simulink model "Hermes"  (R2022a)
settings: Solver=FixedStepAuto  StartTime=0.0  StopTime=10.0  FixedStep=0.005  RelTol=1e-3
values from neighbouring files (symbols this model uses):
  Car_mass = Car_Mass_lb * 0.45359    (= 272.154)    [hermes_physical_parameters.m]    (also in hermes_physical_parameters.mat; input_signals.mat)
  Car_moment_of_inertia = 4 * (0.06631756 + 0.06646249)    (= 0.5311202)    [hermes_physical_parameters.m]    (also in hermes_physical_parameters.mat; input_signals.mat)
  Cross_sectional_area = 0.78    [hermes_physical_parameters.m]    (also in hermes_physical_parameters.mat; input_signals.mat)
  DIFF_ratio = 9    [datasheet.mat]    (also in hermes_system_parameters.m = 8.38; hermes_system_parameters.mat = 8.38; input_signals.mat = 8.38)
  Drag_coeff = 0.5    [datasheet.mat]    (also in hermes_physical_parameters.m = 0.906; hermes_physical_parameters.mat = 0.906; input_signals.mat = 0.906)
  ECVT_angle = 13    [hermes_system_parameters.m]    (also in hermes_system_parameters.mat; input_signals.mat)
  ECVT_clamp_gain = 0.0001    [datasheet.mat]    (also in hermes_system_parameters.m = 0.001; hermes_system_parameters.mat = 0.001; input_signals.mat = 0.0006)
  ECVT_efficiency = 0.8    [datasheet.mat]    (also in hermes_physical_parameters.m = 0.88; hermes_physical_parameters.mat = 0.88; input_signals.mat = 0.88)
  ECVT_friction_coeff = 0.51    [hermes_physical_parameters.m]    (also in hermes_physical_parameters.mat; input_signals.mat)
  ECVT_max_clamp_force = ECVT_max_clamp_force * 4.4482189    (= 889.64378)    [hermes_system_parameters.m]    (also in hermes_system_parameters.mat; input_signals.mat)
  ECVT_MAX_ratio = 4.24    [datasheet.mat]    (also in hermes_system_parameters.m = 4.31; hermes_system_parameters.mat = 4.31; input_signals.mat = 4.31)
  ECVT_MIN_ratio = 0.81    [datasheet.mat]    (also in hermes_system_parameters.m; hermes_system_parameters.mat; input_signals.mat)
  ECVT_P_gain = 7e-05    [datasheet.mat]    (also in hermes_system_parameters.m; hermes_system_parameters.mat; input_signals.mat)
  ECVT_rate_limit = (ECVT_MAX_ratio - ECVT_MIN_ratio) / ECVT_shift_time    (= 3.5)    [hermes_system_parameters.m]    (also in hermes_system_parameters.mat; input_signals.mat)
  Engine_efficiency = 0.9    [datasheet.mat]    (also in hermes_physical_parameters.m = 1; hermes_physical_parameters.mat = 1; input_signals.mat = 1)
  Engine_moment_of_inertia = 0.00172765 + 0.03589500    (= 0.03762265)    [hermes_physical_parameters.m]    (also in hermes_physical_parameters.mat; input_signals.mat)
  GRAVITY = 9.81    [datasheet.mat]    (also in hermes_physical_parameters.m; hermes_physical_parameters.mat; input_signals.mat)
  launch_control_enabled = 1    [input_signals.mat]
  Locked_regime_rpm = 3200    [hermes_system_parameters.m]    (also in hermes_system_parameters.mat; input_signals.mat = 3100)
  Rolling_coeff = 0.125    [hermes_physical_parameters.m]    (also in hermes_physical_parameters.mat; input_signals.mat)
  RPM_MAX = 3600    [datasheet.mat]    (also in hermes_physical_parameters.m; hermes_physical_parameters.mat; input_signals.mat)
  RPM_STALL = 1800    [datasheet.mat]    (also in hermes_physical_parameters.m = 2200; hermes_physical_parameters.mat = 2200; input_signals.mat = 2200)
  Slip_regime_rpm = 2400    [hermes_system_parameters.m]    (also in hermes_system_parameters.mat; input_signals.mat = 2800)
  Torque_regime_limit = 10176    [datasheet.mat]
  Transmission_efficiency = 0.95 * 0.95 * 0.95 * 0.95    (= 0.81450625)    [hermes_physical_parameters.m]    (also in hermes_physical_parameters.mat; input_signals.mat)
  Wheel_radius = 0.2921    [datasheet.mat]    (also in hermes_physical_parameters.m; hermes_physical_parameters.mat; input_signals.mat)
undefined symbols (not defined in the file or in its folder): Target_Engine_rpm, Wheel_RPM
libraries: simulink_extras x3, simulink x1
settings Model: Creator=garyw  LastModifiedBy=garyw

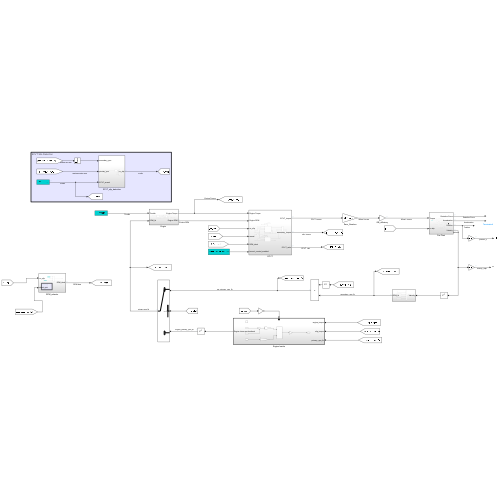
[thumbnail: Simulink's stored preview of the top-level diagram]
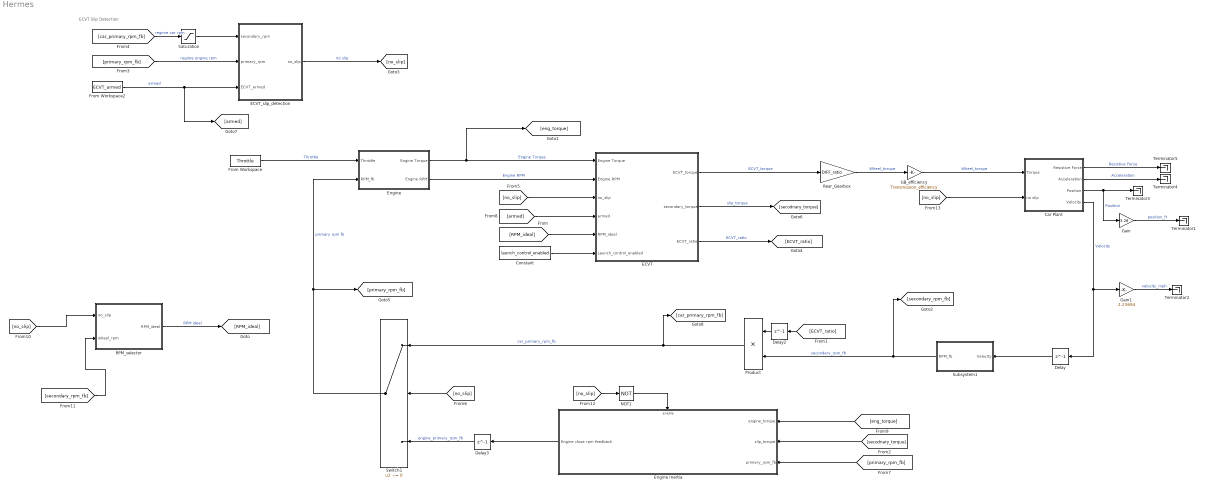
== system Hermes ==
  note: ECVT Slip Detection
  Car Plant : Subsystem
  Constant : Constant  Value=launch_control_enabled
  Delay : Delay  DelayLength=1
  Delay2 : Delay  DelayLength=1  InitialCondition=ECVT_MAX_ratio
  Delay3 : Delay  DelayLength=1  InitialCondition=1800
  ECVT : Subsystem
  ECVT_slip_detection : Subsystem
  Engine : Subsystem
  Engine Inertia : Subsystem
  From Workspace : FromWorkspace  VariableName=Throttle
  From Workspace2 : FromWorkspace  VariableName=ECVT_armed
  GB_efficiency : Gain  Gain=Transmission_efficiency
  Gain : Gain  Gain=3.28
  Gain1 : Gain  Gain=2.23694
  NOT1 : Logic  Operator=NOT  IconShape=distinctive  AllPortsSameDT=off  OutDataTypeStr=boolean
  Product : Product
  RPM_selector : Subsystem
  Rear_Gearbox : Gain  Gain=DIFF_ratio
  Saturation : Saturate  UpperLimit=inf  LowerLimit=0.001
  Subsystem1 : Subsystem
  Switch1 : Switch  Criteria=u2 ~= 0  SaturateOnIntegerOverflow=off  InputSameDT=off
  Terminator{1..5} (5 alike) : Terminator
  wires:
  From Workspace/1 -> Engine/1(Throttle)  "Throttle"
  Engine/1(Engine Torque) -> [eng_torque], ECVT/1(Engine Torque)  "Engine Torque"
  GB_efficiency/1 -> Car Plant/1(Torque)  "Wheel_torque"
  Car Plant/2(Acceleration) -> Terminator4/1  "Acceleration"
  Car Plant/3(Position) -> Terminator3/1, Gain/1  "Position"
  RPM_selector/1(RPM_ideal) -> [RPM_ideal]  "RPM ideal"
  ECVT_slip_detection/1(no_slip) -> [no_slip]  "no slip"
  Subsystem1/1(RPM_fb) -> [secondary_rpm_fb], Product/2  "secondary_rpm_fb"
  Car Plant/4(Velocity) -> Gain1/1, Delay/1  "Velocity"
  [no_slip] -> Switch1/2
  [primary_rpm_fb] -> Engine Inertia/3(primary_rpm_fb)
  [secodnary_torque] -> Engine Inertia/2(slip_torque)
  [eng_torque] -> Engine Inertia/1(engine_torque)
  Switch1/1 -> [primary_rpm_fb], Engine/2(RPM_fb)  "primary rpm fb"
  Product/1 -> [car_primary_rpm_fb], Switch1/1  "car_primary_rpm_fb"
  [ECVT_ratio] -> Delay2/1
  Engine Inertia/1(Engine close rpm feedback) -> Delay3/1
  [no_slip] -> NOT1/1
  NOT1/1 -> Engine Inertia/Enable
  [primary_rpm_fb] -> ECVT_slip_detection/2(primary_rpm)  "regime engine rpm"
  [car_primary_rpm_fb] -> Saturation/1  "regime car rpm"
  Delay/1 -> Subsystem1/1(Velocity)
  Saturation/1 -> ECVT_slip_detection/1(secondary_rpm)
  Delay2/1 -> Product/1
  Delay3/1 -> Switch1/3  "engine_primary_rpm_fb"
  [no_slip] -> Car Plant/2(no slip)
  From Workspace2/1 -> [armed], ECVT_slip_detection/3(ECVT_armed)  "armed"
  Engine/2(Engine RPM) -> ECVT/2(Engine RPM)  "Engine RPM"
  ECVT/1(ECVT_torque) -> Rear_Gearbox/1  "ECVT_torque"
  [RPM_ideal] -> ECVT/5(RPM_ideal)
  ECVT/3(ECVT_ratio) -> [ECVT_ratio]  "ECVT_ratio"
  ECVT/2(secondary_torque) -> [secodnary_torque]  "slip_torque"
  [no_slip] -> ECVT/3(no_slip)
  [armed] -> ECVT/4(armed)
  Rear_Gearbox/1 -> GB_efficiency/1  "Wheel_torque"
  [no_slip] -> RPM_selector/1(no_slip)
  Constant/1 -> ECVT/6(Launch_control_enabled)
  Gain/1 -> Terminator1/1  "position_ft"
  Gain1/1 -> Terminator2/1  "velocity_mph"
  [secondary_rpm_fb] -> RPM_selector/2(wheel_rpm)
  Car Plant/1(Resistive Force) -> Terminator5/1  "Resistive Force"

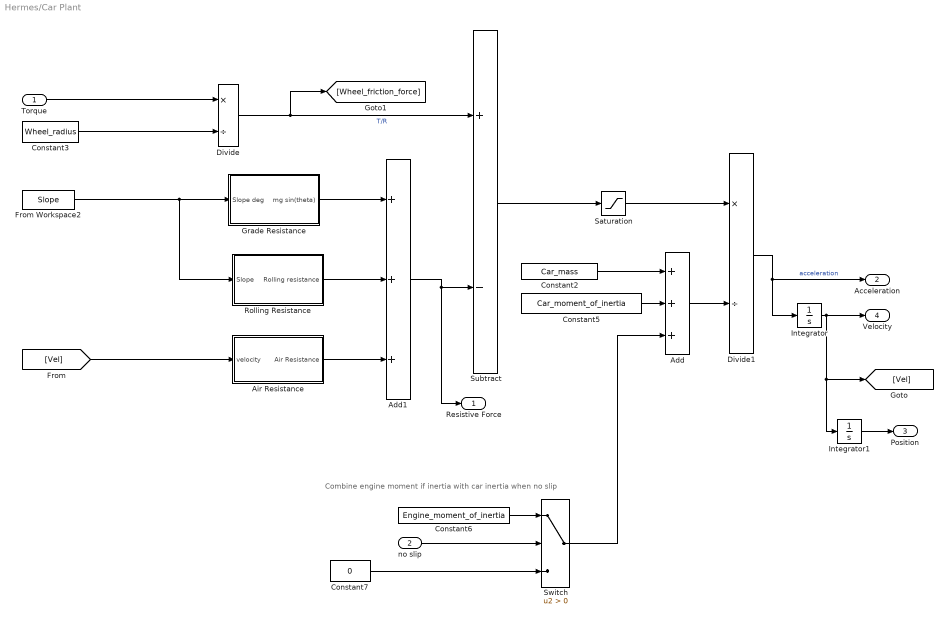
== system Hermes/Car Plant ==
  note: Combine engine moment if inertia with car inertia when no slip
  Torque : Inport
  no slip : Inport  Port=2
  Add : Sum  Inputs=+++
  Add1 : Sum  Inputs=+++
  Air Resistance : Subsystem
  Constant2 : Constant  Value=Car_mass
  Constant3 : Constant  Value=Wheel_radius
  Constant5 : Constant  Value=Car_moment_of_inertia
  Constant6 : Constant  Value=Engine_moment_of_inertia
  Constant7 : Constant  Value=0
  Divide : Product  Inputs=*/
  Divide1 : Product  Inputs=*/
  From Workspace2 : FromWorkspace  VariableName=Slope
  Grade Resistance : Subsystem
  Integrator : Integrator
  Integrator1 : Integrator
  Rolling Resistance : Subsystem
  Saturation : Saturate  UpperLimit=inf  LowerLimit=0
  Subtract : Sum  Inputs=+-
  Switch : Switch  Criteria=u2 > Threshold  SaturateOnIntegerOverflow=off  InputSameDT=off
  Resistive Force : Outport
  Acceleration : Outport  Port=2
  Position : Outport  Port=3
  Velocity : Outport  Port=4
  wires:
  Constant3/1 -> Divide/2
  Divide/1 -> [Wheel_friction_force], Subtract/1  "T/R"
  Subtract/1 -> Saturation/1
  Divide1/1 -> Integrator/1, Acceleration/1  "acceleration"
  Torque/1 -> Divide/1
  Integrator/1 -> [Vel], Integrator1/1, Velocity/1
  Integrator1/1 -> Position/1
  Constant2/1 -> Add/1
  Add/1 -> Divide1/2
  Constant5/1 -> Add/2
  Switch/1 -> Add/3
  Constant6/1 -> Switch/1
  no slip/1 -> Switch/2
  Constant7/1 -> Switch/3
  From Workspace2/1 -> Rolling Resistance/1(Slope), Grade Resistance/1(Slope deg)
  Grade Resistance/1(mg sin(theta)) -> Add1/1
  [Vel] -> Air Resistance/1(velocity)
  Rolling Resistance/1(Rolling resistance) -> Add1/2
  Air Resistance/1(Air Resistance) -> Add1/3
  Saturation/1 -> Divide1/1
  Add1/1 -> Resistive Force/1, Subtract/2

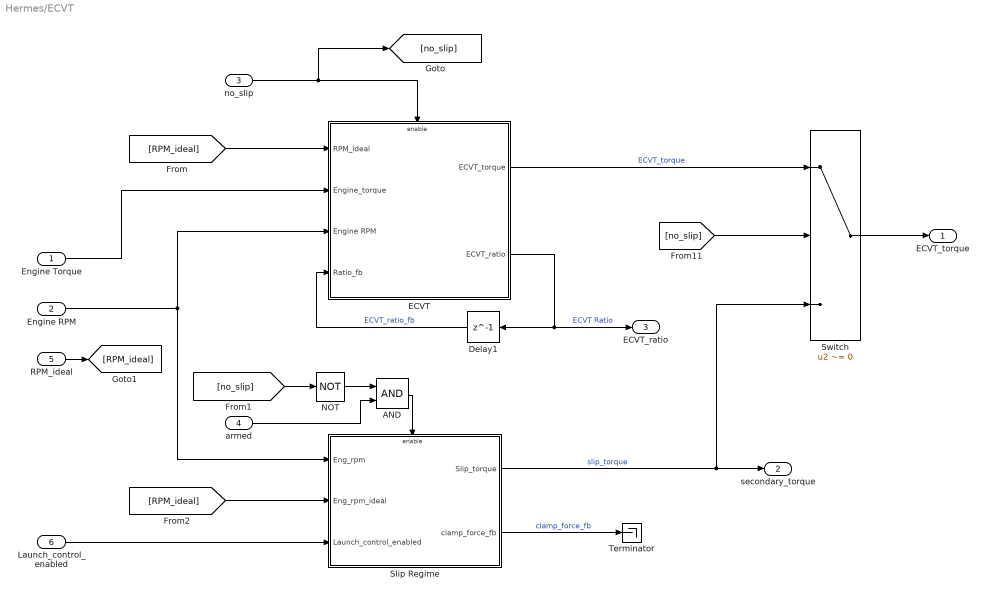
== system Hermes/ECVT ==
  Engine Torque : Inport
  Engine RPM : Inport  Port=2
  no_slip : Inport  Port=3
  armed : Inport  Port=4
  RPM_ideal : Inport  Port=5
  Launch_control_enabled : Inport  Port=6
  AND : Logic  AllPortsSameDT=off  OutDataTypeStr=boolean
  Delay1 : Delay  DelayLength=1  InitialCondition=ECVT_MAX_ratio
  ECVT : Subsystem
  NOT : Logic  Operator=NOT  IconShape=distinctive  AllPortsSameDT=off  OutDataTypeStr=boolean
  Slip Regime : Subsystem
  Switch : Switch  Criteria=u2 ~= 0  SaturateOnIntegerOverflow=off  InputSameDT=off
  Terminator : Terminator
  ECVT_torque : Outport
  secondary_torque : Outport  Port=2
  ECVT_ratio : Outport  Port=3
  wires:
  [RPM_ideal] -> Slip Regime/2(Eng_rpm_ideal)
  ECVT/1(ECVT_torque) -> Switch/1  "ECVT_torque"
  [RPM_ideal] -> ECVT/1(RPM_ideal)
  Slip Regime/1(Slip_torque) -> secondary_torque/1, Switch/3  "slip_torque"
  Delay1/1 -> ECVT/4(Ratio_fb)  "ECVT_ratio_fb"
  Engine RPM/1 -> Slip Regime/1(Eng_rpm), ECVT/3(Engine RPM)
  no_slip/1 -> [no_slip], ECVT/Enable
  [no_slip] -> NOT/1
  ECVT/2(ECVT_ratio) -> ECVT_ratio/1, Delay1/1  "ECVT Ratio"
  NOT/1 -> AND/1
  [no_slip] -> Switch/2
  Slip Regime/2(clamp_force_fb) -> Terminator/1  "clamp_force_fb"
  AND/1 -> Slip Regime/Enable
  armed/1 -> AND/2
  Engine Torque/1 -> ECVT/2(Engine_torque)
  Switch/1 -> ECVT_torque/1
  RPM_ideal/1 -> [RPM_ideal]
  Launch_control_enabled/1 -> Slip Regime/3(Launch_control_enabled)

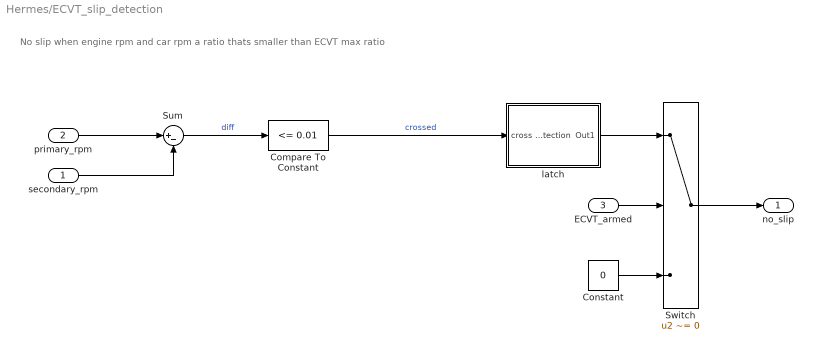
== system Hermes/ECVT_slip_detection ==
  note: No slip when engine rpm and car rpm a ratio thats smaller than ECVT max ratio
  secondary_rpm : Inport
  primary_rpm : Inport  Port=2
  ECVT_armed : Inport  Port=3
  Compare To Constant : simulink/Logic and Bit Operations/Compare To Constant  relop=<=  const=0.01  OutDataTypeStr=boolean
  Constant : Constant  Value=0
  Sum : Sum  Inputs=|+-
  Switch : Switch  Criteria=u2 ~= 0  SaturateOnIntegerOverflow=off  InputSameDT=off
  latch : Subsystem
  no_slip : Outport
  wires:
  secondary_rpm/1 -> Sum/2
  primary_rpm/1 -> Sum/1
  Compare To Constant/1 -> latch/1(cross detection)  "crossed"
  Sum/1 -> Compare To Constant/1  "diff"
  Switch/1 -> no_slip/1
  Constant/1 -> Switch/3
  ECVT_armed/1 -> Switch/2
  latch/1(Out1) -> Switch/1

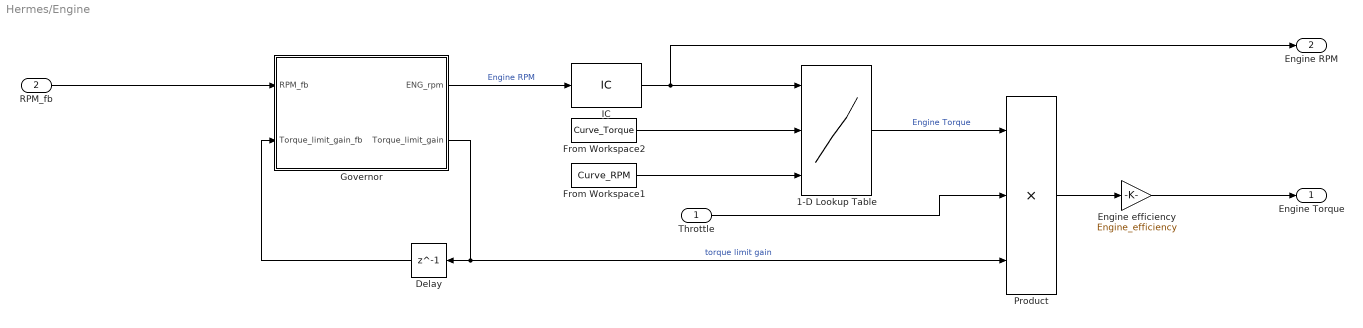
== system Hermes/Engine ==
  Throttle : Inport
  RPM_fb : Inport  Port=2
  1-D Lookup Table : Lookup_n-D  NumberOfTableDimensions=1  BreakpointsForDimension1Source=Input port  BreakpointsForDimension1=[-5:5]  TableSource=Input port  Table=tanh([-5:5])  InternalRulePriority=Speed  RndMeth=Simplest
      settings: InputPortMap=u0,p221,p5
  Delay : Delay  DelayLength=1  InitialCondition=1
  Engine efficiency : Gain  Gain=Engine_efficiency
  From Workspace1 : FromWorkspace  VariableName=Curve_RPM
  From Workspace2 : FromWorkspace  VariableName=Curve_Torque
  Governor : Subsystem
  IC : InitialCondition  Value=1800
  Product : Product  Inputs=3
  Engine Torque : Outport
  Engine RPM : Outport  Port=2
  wires:
  From Workspace2/1 -> 1-D Lookup Table/2
  From Workspace1/1 -> 1-D Lookup Table/3
  1-D Lookup Table/1 -> Product/1  "Engine Torque"
  IC/1 -> Engine RPM/1, 1-D Lookup Table/1
  Governor/2(Torque_limit_gain) -> Product/3, Delay/1  "torque limit gain"
  Delay/1 -> Governor/2(Torque_limit_gain_fb)
  Product/1 -> Engine efficiency/1
  Throttle/1 -> Product/2
  Engine efficiency/1 -> Engine Torque/1
  RPM_fb/1 -> Governor/1(RPM_fb)
  Governor/1(ENG_rpm) -> IC/1  "Engine RPM"

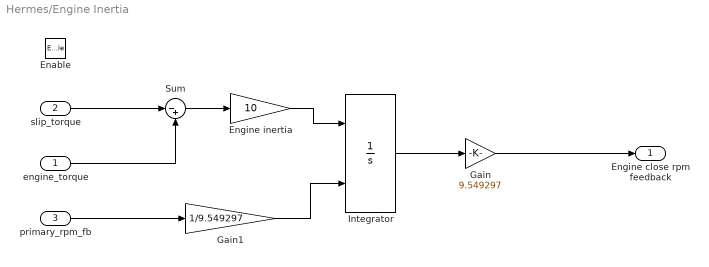
== system Hermes/Engine Inertia ==
  engine_torque : Inport
  slip_torque : Inport  Port=2
  primary_rpm_fb : Inport  Port=3
  Enable : EnablePort
  Engine inertia : Gain  Gain=10
  Gain : Gain  Gain=9.549297
  Gain1 : Gain  Gain=1/9.549297
  Integrator : Integrator  InitialConditionSource=external
  Sum : Sum  Inputs=|-+
  Engine close rpm feedback : Outport
  wires:
  primary_rpm_fb/1 -> Gain1/1
  slip_torque/1 -> Sum/1
  Sum/1 -> Engine inertia/1
  Engine inertia/1 -> Integrator/1
  engine_torque/1 -> Sum/2
  Integrator/1 -> Gain/1
  Gain/1 -> Engine close rpm feedback/1
  Gain1/1 -> Integrator/2

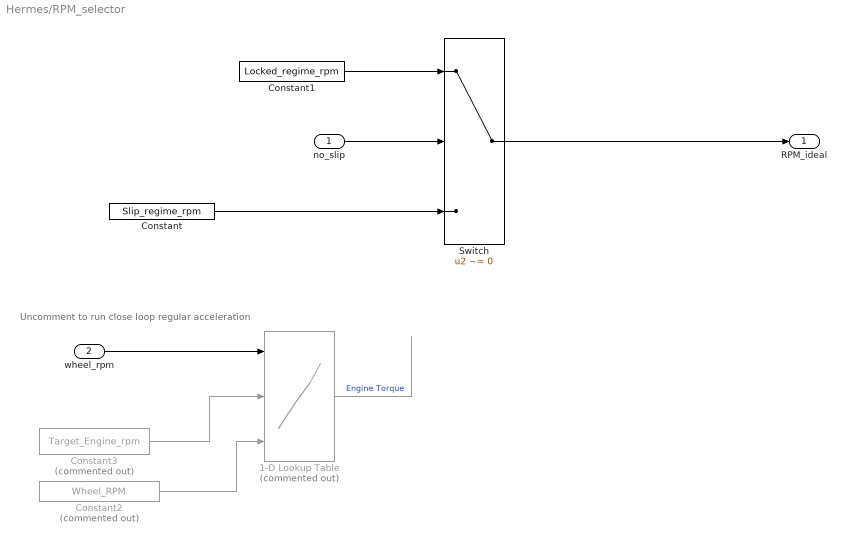
== system Hermes/RPM_selector ==
  note: Uncomment to run close loop regular acceleration
  no_slip : Inport
  wheel_rpm : Inport  Port=2
  1-D Lookup Table : Lookup_n-D  Commented=on  NumberOfTableDimensions=1  BreakpointsForDimension1Source=Input port  BreakpointsForDimension1=[-5:5]  TableSource=Input port  Table=tanh([-5:5])  InternalRulePriority=Speed  RndMeth=Simplest
      settings: InputPortMap=u0,p221,p5
  Constant : Constant  Value=Slip_regime_rpm
  Constant1 : Constant  Value=Locked_regime_rpm
  Constant2 : Constant  Commented=on  Value=Wheel_RPM
  Constant3 : Constant  Commented=on  Value=Target_Engine_rpm
  Switch : Switch  Criteria=u2 ~= 0  Threshold=Torque_regime_limit  SaturateOnIntegerOverflow=off  InputSameDT=off
  RPM_ideal : Outport
  wires:
  Constant/1 -> Switch/3
  Constant1/1 -> Switch/1
  Switch/1 -> RPM_ideal/1
  no_slip/1 -> Switch/2
  wheel_rpm/1 -> 1-D Lookup Table/1
  Constant3/1 -> 1-D Lookup Table/2
  Constant2/1 -> 1-D Lookup Table/3
  1-D Lookup Table/1 -> ?  "Engine Torque"

== system Hermes/Subsystem1 ==
  Velocity : Inport
  Constant : Constant  Value=Wheel_radius
  Constant1 : Constant  Value=DIFF_ratio
  Divide1 : Product  Inputs=**/*
  rad/s to RPM : Constant  Value=9.549297
  RPM_fb : Outport
  wires:
  Divide1/1 -> RPM_fb/1  "RPM_fb"
  Constant/1 -> Divide1/3
  rad/s to RPM/1 -> Divide1/2
  Constant1/1 -> Divide1/4
  Velocity/1 -> Divide1/1

== system Hermes/Car Plant/Air Resistance ==
  velocity : Inport
  Constant : Constant  Value=Cross_sectional_area
  Constant1 : Constant  Value=0.5
  Constant4 : Constant  Value=Drag_coeff
  Product2 : Product  Inputs=4
  Square : Math  Operator=square
  Air Resistance : Outport
  wires:
  Constant4/1 -> Product2/1
  velocity/1 -> Square/1
  Product2/1 -> Air Resistance/1
  Square/1 -> Product2/2
  Constant/1 -> Product2/3
  Constant1/1 -> Product2/4

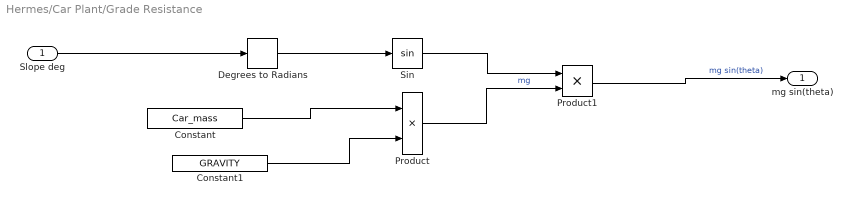
== system Hermes/Car Plant/Grade Resistance ==
  Slope deg : Inport
  Constant : Constant  Value=Car_mass
  Constant1 : Constant  Value=GRAVITY
  Degrees to Radians : simulink_extras/Transformations/Degrees to Radians
  Product : Product
  Product1 : Product
  Sin : Trigonometry
  mg sin(theta) : Outport
  wires:
  Product/1 -> Product1/2  "mg"
  Sin/1 -> Product1/1
  Product1/1 -> mg sin(theta)/1  "mg sin(theta)"
  Constant/1 -> Product/1
  Slope deg/1 -> Degrees to Radians/1
  Constant1/1 -> Product/2
  Degrees to Radians/1 -> Sin/1

== system Hermes/Car Plant/Rolling Resistance ==
  Slope : Inport
  Abs : Abs  SaturateOnIntegerOverflow=off
  Constant : Constant  Value=Rolling_coeff
  Constant1 : Constant  Value=Car_mass
  Cos : Trigonometry  Operator=cos
  Degrees to Radians : simulink_extras/Transformations/Degrees to Radians
  Product : Product  Inputs=3
  Rolling resistance : Outport
  wires:
  Slope/1 -> Degrees to Radians/1
  Degrees to Radians/1 -> Cos/1
  Cos/1 -> Product/3
  Constant1/1 -> Product/2
  Constant/1 -> Product/1
  Product/1 -> Abs/1
  Abs/1 -> Rolling resistance/1

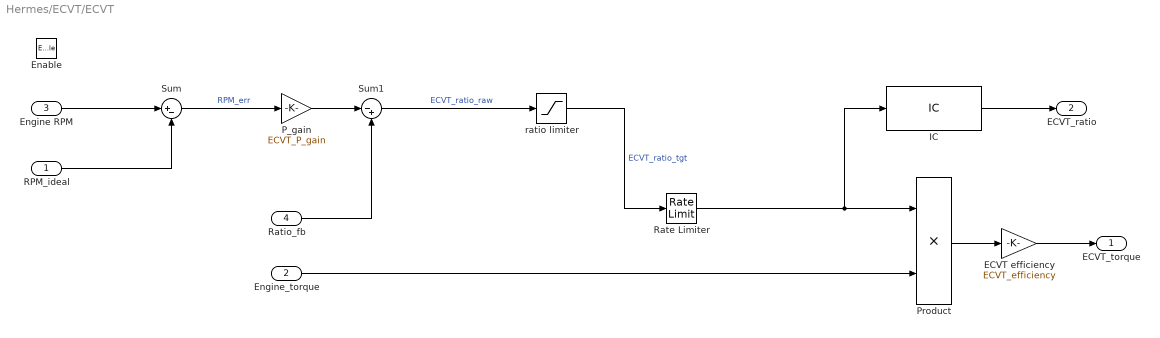
== system Hermes/ECVT/ECVT ==
  RPM_ideal : Inport
  Engine_torque : Inport  Port=2
  Engine RPM : Inport  Port=3
  Ratio_fb : Inport  Port=4
  Enable : EnablePort
  ECVT efficiency : Gain  Gain=ECVT_efficiency
  IC : InitialCondition  Value=ECVT_MAX_ratio
  P_gain : Gain  Gain=ECVT_P_gain
  Product : Product
  Rate Limiter : RateLimiter  RisingSlewLimit=ECVT_rate_limit  FallingSlewLimit=-ECVT_rate_limit  SampleTimeMode=inherited
  Sum : Sum  Inputs=|+-
  Sum1 : Sum  Inputs=|-+
  ratio limiter : Saturate  UpperLimit=ECVT_MAX_ratio  LowerLimit=ECVT_MIN_ratio
  ECVT_torque : Outport
  ECVT_ratio : Outport  Port=2
  wires:
  Engine RPM/1 -> Sum/1
  RPM_ideal/1 -> Sum/2
  Sum/1 -> P_gain/1  "RPM_err"
  P_gain/1 -> Sum1/1
  Ratio_fb/1 -> Sum1/2
  Sum1/1 -> ratio limiter/1  "ECVT_ratio_raw"
  Engine_torque/1 -> Product/2
  Product/1 -> ECVT efficiency/1
  ECVT efficiency/1 -> ECVT_torque/1
  IC/1 -> ECVT_ratio/1
  ratio limiter/1 -> Rate Limiter/1  "ECVT_ratio_tgt"
  Rate Limiter/1 -> IC/1, Product/1

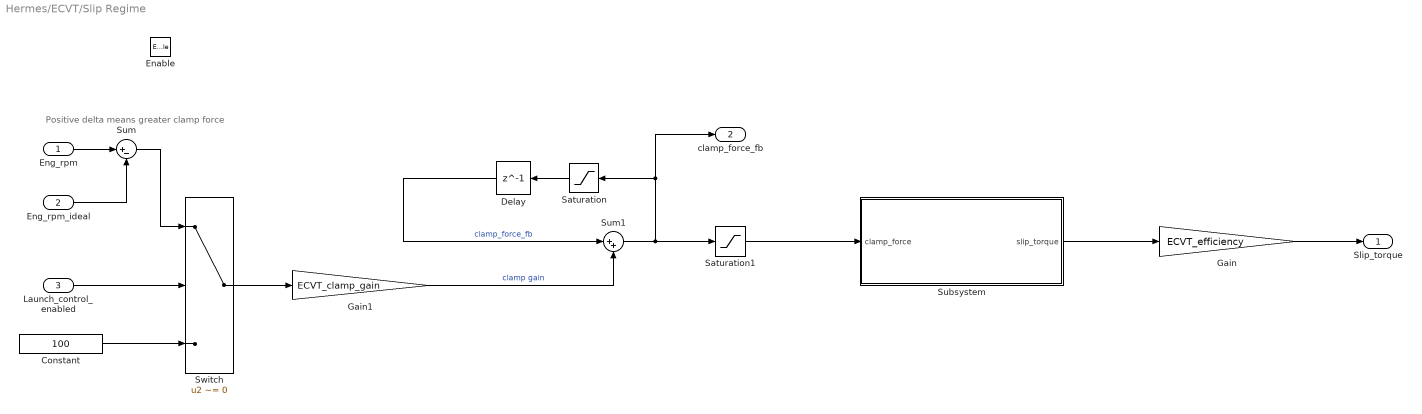
== system Hermes/ECVT/Slip Regime ==
  note: Positive delta means greater clamp force
  Eng_rpm : Inport
  Eng_rpm_ideal : Inport  Port=2
  Launch_control_enabled : Inport  Port=3
  Enable : EnablePort
  Constant : Constant  Value=100
  Delay : Delay  DelayLength=1  InitialCondition=0
  Gain : Gain  Gain=ECVT_efficiency
  Gain1 : Gain  Gain=ECVT_clamp_gain
  Saturation : Saturate  UpperLimit=inf  LowerLimit=0
  Saturation1 : Saturate  UpperLimit=ECVT_max_clamp_force  LowerLimit=0
  Subsystem : Subsystem
  Sum : Sum  Inputs=|+-
  Sum1 : Sum  Inputs=|++
  Switch : Switch  Criteria=u2 ~= 0  SaturateOnIntegerOverflow=off  InputSameDT=off
  Slip_torque : Outport
  clamp_force_fb : Outport  Port=2
  wires:
  Eng_rpm_ideal/1 -> Sum/2
  Eng_rpm/1 -> Sum/1
  Sum/1 -> Switch/1
  Gain1/1 -> Sum1/2  "clamp gain"
  Sum1/1 -> Saturation1/1, clamp_force_fb/1, Saturation/1
  Delay/1 -> Sum1/1  "clamp_force_fb"
  Subsystem/1(slip_torque) -> Gain/1
  Saturation/1 -> Delay/1
  Gain/1 -> Slip_torque/1
  Saturation1/1 -> Subsystem/1(clamp_force)
  Launch_control_enabled/1 -> Switch/2
  Constant/1 -> Switch/3
  Switch/1 -> Gain1/1

== system Hermes/ECVT_slip_detection/latch ==
  cross detection : Inport
  Delay : Delay  DelayLength=1
  Switch : Switch  Criteria=u2 ~= 0  SaturateOnIntegerOverflow=off  InputSameDT=off
  Out1 : Outport
  wires:
  cross detection/1 -> Switch/2, Switch/1
  Switch/1 -> Delay/1, Out1/1
  Delay/1 -> Switch/3

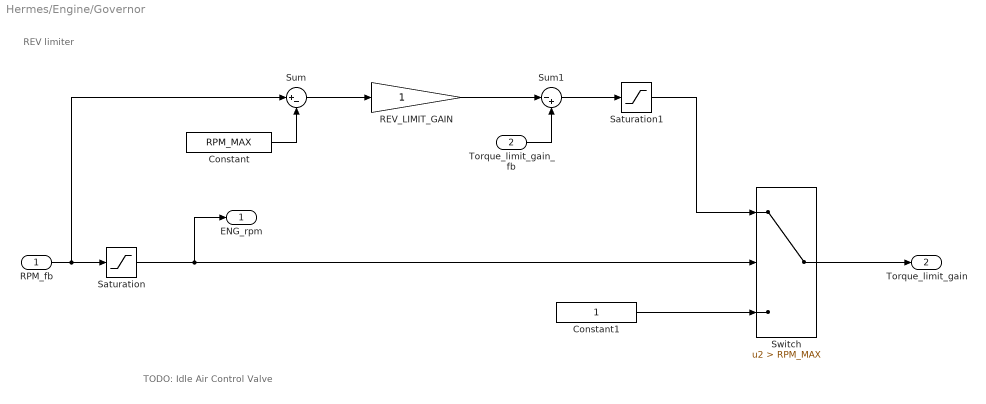
== system Hermes/Engine/Governor ==
  note: REV limiter
  note: TODO: Idle Air Control Valve
  RPM_fb : Inport
  Torque_limit_gain_fb : Inport  Port=2
  Constant : Constant  Value=RPM_MAX
  Constant1 : Constant
  REV_LIMIT_GAIN : Gain
  Saturation : Saturate  UpperLimit=inf  LowerLimit=RPM_STALL
  Saturation1 : Saturate  UpperLimit=1  LowerLimit=0
  Sum : Sum  Inputs=|+-
  Sum1 : Sum  Inputs=|-+
  Switch : Switch  Criteria=u2 > Threshold  Threshold=RPM_MAX  SaturateOnIntegerOverflow=off  InputSameDT=off
  ENG_rpm : Outport
  Torque_limit_gain : Outport  Port=2
  wires:
  RPM_fb/1 -> Sum/1, Saturation/1
  Saturation/1 -> Switch/2, ENG_rpm/1
  Constant/1 -> Sum/2
  Sum/1 -> REV_LIMIT_GAIN/1
  REV_LIMIT_GAIN/1 -> Sum1/1
  Torque_limit_gain_fb/1 -> Sum1/2
  Sum1/1 -> Saturation1/1
  Saturation1/1 -> Switch/1
  Switch/1 -> Torque_limit_gain/1
  Constant1/1 -> Switch/3

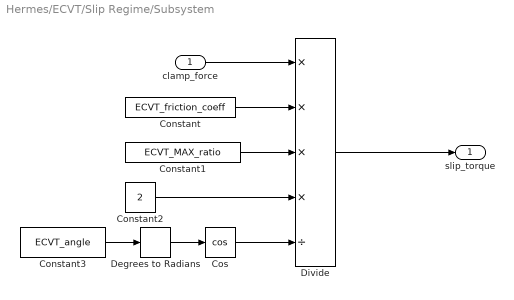
== system Hermes/ECVT/Slip Regime/Subsystem ==
  clamp_force : Inport
  Constant : Constant  Value=ECVT_friction_coeff
  Constant1 : Constant  Value=ECVT_MAX_ratio
  Constant2 : Constant  Value=2
  Constant3 : Constant  Value=ECVT_angle
  Cos : Trigonometry  Operator=cos
  Degrees to Radians : simulink_extras/Transformations/Degrees to Radians
  Divide : Product  Inputs=****/
  slip_torque : Outport
  wires:
  clamp_force/1 -> Divide/1
  Constant/1 -> Divide/2
  Constant1/1 -> Divide/3
  Constant2/1 -> Divide/4
  Constant3/1 -> Degrees to Radians/1
  Degrees to Radians/1 -> Cos/1
  Cos/1 -> Divide/5
  Divide/1 -> slip_torque/1
